simulink library "steeringWheel_lib"  (R2022b)
settings: Solver=VariableStepAuto  StartTime=0.0  StopTime=10.0  RelTol=1e-3
undefined symbols (not defined in the file): raptor_xcp_function
libraries: Raptor_lib x6
settings Model: Creator=serga  LastModifiedBy=serga

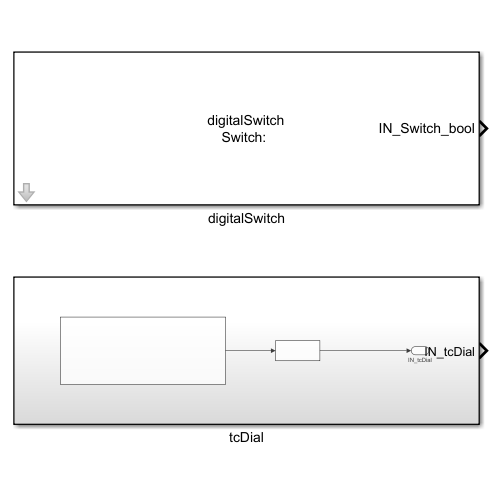
[thumbnail: Simulink's stored preview of the top-level diagram]
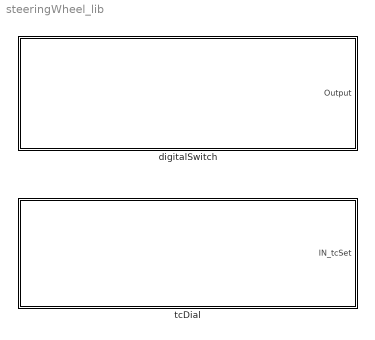
== system steeringWheel_lib ==
  digitalSwitch : Subsystem  mask{pos=''}
      mask prompts: pos "Position"
      mask Display:
      | disp(['digitalSwitch\n'...
      |     'Switch: ' pos]);
      | port_label('output', 1, ['IN_' pos 'Switch_bool']);
  tcDial : Subsystem

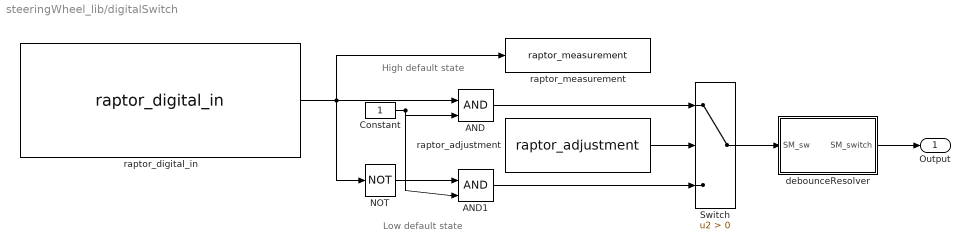
== system steeringWheel_lib/digitalSwitch ==
  note: Low default state
  note: High default state
  AND : Logic  IconShape=distinctive  AllPortsSameDT=off  OutDataTypeStr=boolean
  AND1 : Logic  IconShape=distinctive  AllPortsSameDT=off  OutDataTypeStr=boolean
  Constant : Constant
  NOT : Logic  Operator=NOT  IconShape=distinctive  AllPortsSameDT=off  OutDataTypeStr=boolean
  Switch : Switch  Criteria=u2 > Threshold  SaturateOnIntegerOverflow=off  InputSameDT=off
  debounceResolver : Stateflow chart  TreatAsAtomicUnit=on
  raptor_adjustment : Raptor_lib/Data Storage/raptor_adjustment  paramName=['IN_' pos 'PolarityOverride_bool']  nameSource=Parameter  initValue=0.00  dataType=boolean  storage=Calibration  calDispType=Number  calEnum={'False', 'True'}  calGain=1.0  calOffset=0.0  calMax=inf  calMin=-inf  calFormat='-1'  calUnit=''  calHelp=''  calAccess=1  calFunction=raptor_xcp_function(gcb)  calDispHeaders=off  calColHeaders={'Col1' 'Col2' 'Col3'}  calRowHeaders={'Row1' 'Row2' 'Row3'}
      settings: SourceProductName=Raptor
  raptor_digital_in : Raptor_lib/Input & Output/raptor_digital_in  resourceValues=WAKE_INPUT1|INPUT33|INPUT34|INPUT35|INPUT36|INPUT37|INPUT38|INPUT39|INPUT40|(None)  resource=INPUT33  pullUDValues=1.3k PD  pullUD=1.3k PD  upperThres='RAPTOR MASK DEFAULT'  lowerThres='RAPTOR MASK DEFAULT'
      settings: SourceProductName=Raptor
  raptor_measurement : Raptor_lib/Data Storage/raptor_measurement  paramName=['IN_' pos 'Polarity_bool']  nameSource=Parameter  calDispType=Number  calEnum={'False', 'True'}  calGain=1.0  calOffset=0.0  calMax=inf  calMin=-inf  calFormat='-1'  calUnit=''  calHelp=''  calAccess=1  calFunction=raptor_xcp_function(gcb)  calVisible=on
      settings: SourceProductName=Raptor
  Output : Outport
  wires:
  raptor_digital_in/1 -> raptor_measurement/1, NOT/1, AND/1
  Constant/1 -> AND1/2, AND/2
  NOT/1 -> AND1/1
  AND/1 -> Switch/1
  AND1/1 -> Switch/3
  Switch/1 -> debounceResolver/1(SM_sw)
  raptor_adjustment/1 -> Switch/2
  debounceResolver/1(SM_switch) -> Output/1

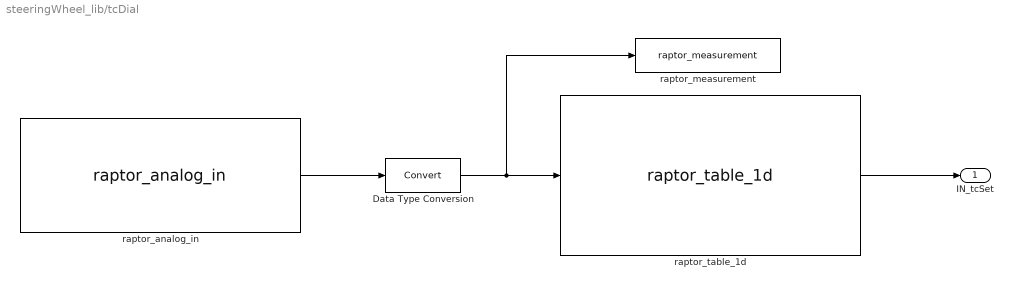
== system steeringWheel_lib/tcDial ==
  Data Type Conversion : DataTypeConversion  SaturateOnIntegerOverflow=off  RndMeth=Floor
  raptor_analog_in : Raptor_lib/Input & Output/raptor_analog_in  resourceValues=[]  resource=INPUT3  rangeValues=0 - 5 V  range=0 - 5 V  filterrateValues=[]  filterrate='RAPTOR MASK DEFAULT'  resolutionValues=[]  resolution=[]  pullUDValues=2.15k PU  pullUD=2.15k PU
      settings: SourceProductName=Raptor
  raptor_measurement : Raptor_lib/Data Storage/raptor_measurement  paramName='IN_tcSetInput'  nameSource=Parameter  calDispType=Number  calEnum={'False', 'True'}  calGain=1.0  calOffset=0.0  calMax=inf  calMin=-inf  calFormat='-1'  calUnit=''  calHelp=''  calAccess=1  calFunction=raptor_xcp_function(gcb)  calVisible=on
      settings: SourceProductName=Raptor
  raptor_table_1d : Raptor_lib/Table Lookup/raptor_table_1d  dataName='IN_tcSetTable'  initValue=[11 10 9 8 7 6 5 4 3 2 1 -1]  dataType=single  storage=Calibration  initValueX=[390 790 1190 1580 1970 2360 3000 3400 3790 4190 4590 4990]  dataTypeXY=single  storageXY=Calibration  calVisible=on  showTable=on  calGain=1.0  calOffset=0.0  calMax=Inf  calMin=-Inf  calFormat='-1'  calUnit='tcSet'  calHelp=''  showBreakpoint=on  dataNameX=[]  calGainX=1.0  calOffsetX=0.0  calMaxX=Inf  calMinX=-Inf  calFormatX='-1'  calUnitX='mV'  calHelpX=''  calAccess=1  calFunction=raptor_xcp_function(gcb)  measureEnable=off  mName=['Data1D_Output']
      settings: SourceProductName=Raptor
  IN_tcSet : Outport
  wires:
  raptor_analog_in/1 -> Data Type Conversion/1
  Data Type Conversion/1 -> raptor_measurement/1, raptor_table_1d/1
  raptor_table_1d/1 -> IN_tcSet/1

== stateflow chart steeringWheel_lib/digitalSwitch/debounceResolver ==
  state Off
    ex: SM_switch = 0;
  state On
    ex: SM_switch = 1;
  (default) -> Off
  On -> Off : [duration(SM_sw < 1) > 0.01]
  Off -> On : [duration(SM_sw >= 0) > 0.01]
  data: SM_sw input; SM_switch output
